simulink model "TVModel_2022"  (R2022a)
settings: Solver=FixedStepDiscrete  StartTime=0.0  StopTime=10.0  FixedStep=0.01  MaxStep=0.01  RelTol=1e-3  EnableMultiTasking=on
undefined symbols (not defined in the file or in its folder): TV
libraries: simulink x5, simulink_extras x4, dspstat3 x2, sharedTrackingLibrary x1, slpidlib x1, eeGeneralControl x1
(part 1 of 4)
settings Model: Creator=giuse  LastModifiedBy=Daniele
settings SolverCC: AutoInsertRateTranBlk=on
settings OptimizationCC: DefaultParameterBehavior=Inlined  UseDivisionForNetSlopeComputation=on  GainParamInheritBuiltInType=on  UseFloatMulNetSlope=on  InlineInvariantSignals=on  PassReuseOutputArgsAs=Individual arguments  ZeroExternalMemoryAtStartup=off  ZeroInternalMemoryAtStartup=off  NoFixptDivByZeroProtection=on  EfficientFloat2IntCast=on  LifeSpan=1  OptimizeBlockOrder=speed  DifferentSizesBufferReuse=on  EfficientTunableParamExpr=on
settings DebuggingCC: ParameterTunabilityLossMsg=error  UnconnectedInputMsg=warning  UnconnectedOutputMsg=warning  UnconnectedLineMsg=warning
settings HardwareCC: ProdBitPerPointer=32  ProdBitPerSizeT=32  ProdBitPerPtrDiffT=32  ProdLargestAtomicInteger=Long  ProdLargestAtomicFloat=Double  ProdWordSize=32  ProdLongLongMode=on  ProdHWDeviceType=ARM Compatible->ARM Cortex-M
settings SFSimCC: SimCustomHeaderCode="#include \"ITB_Nucleo_configuration\\Inc\\acados_wrapper.h\""  SimUserSources=ITB_Nucleo_configuration\Src\acados_wrapper.c  MATLABDynamicMemAlloc=off  CustomCodeUndefinedFunction=DoNotDetect
settings RTWCC: SystemTargetFile=ert.tlc  GenCodeOnly=on  TemplateMakefile=ert_default_tmf  RTWUseSimCustomCode=on  CustomHeaderCode="#include \"ITB_Nucleo_configuration\\Inc\\acados_wrapper.h\""  CustomSource=ITB_Nucleo_configuration\Src\acados_wrapper.c  DLArmComputeVersion=19.05
settings CodeAppCC: ForceParamTrailComments=on  IgnoreCustomStorageClasses=off  OperatorAnnotations=on  SimulinkDataObjDesc=on  SFDataObjDesc=on  CustomSymbolStrGlobalVar=rt$N$M  CustomSymbolStrType=$N$M  CustomSymbolStrFcn=$N$M$F  CustomSymbolStrMacro=$N$M  InsertBlockDesc=on
settings ERTTargetCC: TargetLangStandard=C99 (ISO)  GenerateSampleERTMain=on  IncludeMdlTerminateFcn=off  CombineSignalStateStructs=on  SuppressErrorStatus=on  SupportAbsoluteTime=off  SupportComplex=off  InlinedParameterPlacement=NonHierarchical  ERTCustomFileTemplate=example_file_process.tlc  ERTFilePackagingFormat=CompactWithDataFile

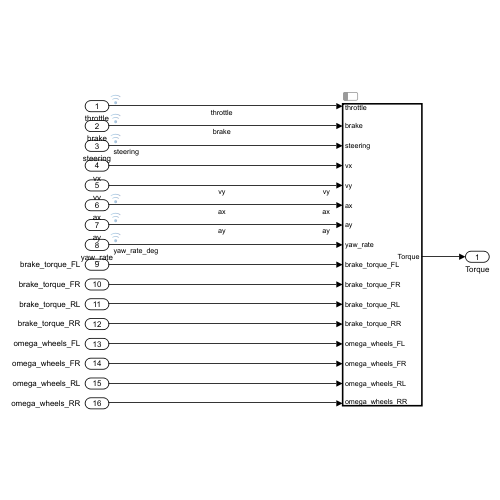
[thumbnail: Simulink's stored preview of the top-level diagram]
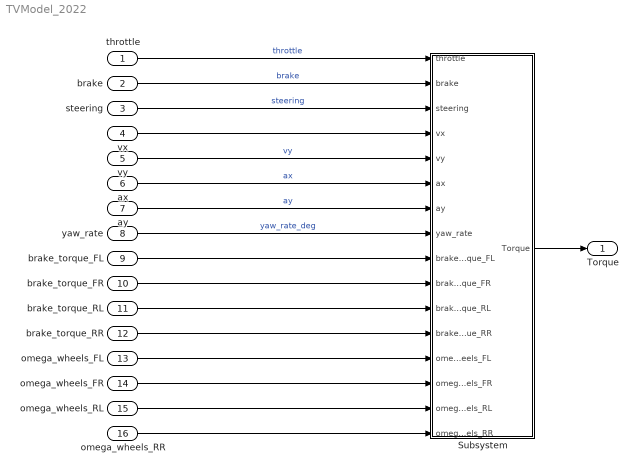
== system TVModel_2022 ==
  throttle : Inport  PortDimensions=1
  brake : Inport  Port=2  PortDimensions=1
  steering : Inport  Port=3  PortDimensions=1
  vx : Inport  Port=4  PortDimensions=1
  vy : Inport  Port=5  PortDimensions=1
  ax : Inport  Port=6  PortDimensions=1
  ay : Inport  Port=7  PortDimensions=1
  yaw_rate : Inport  Port=8  PortDimensions=1
  brake_torque_FL : Inport  Port=9  PortDimensions=1
  brake_torque_FR : Inport  Port=10  PortDimensions=1
  brake_torque_RL : Inport  Port=11  PortDimensions=1
  brake_torque_RR : Inport  Port=12  PortDimensions=1
  omega_wheels_FL : Inport  Port=13  PortDimensions=1
  omega_wheels_FR : Inport  Port=14  PortDimensions=1
  omega_wheels_RL : Inport  Port=15  PortDimensions=1
  omega_wheels_RR : Inport  Port=16  PortDimensions=1
  Subsystem : Subsystem  TreatAsAtomicUnit=on  ScheduleAs=Periodic partition  PartitionName=Subsystem  SystemSampleTime=0.02
  Torque : Outport
  wires:
  vy/1 -> Subsystem/5(vy)  "vy"
  ax/1 -> Subsystem/6(ax)  "ax"
  brake/1 -> Subsystem/2(brake)  "brake"
  ay/1 -> Subsystem/7(ay)  "ay"
  brake_torque_RL/1 -> Subsystem/11(brake_torque_RL)
  brake_torque_RR/1 -> Subsystem/12(brake_torque_RR)
  omega_wheels_RR/1 -> Subsystem/16(omega_wheels_RR)
  omega_wheels_FL/1 -> Subsystem/13(omega_wheels_FL)
  brake_torque_FR/1 -> Subsystem/10(brake_torque_FR)
  yaw_rate/1 -> Subsystem/8(yaw_rate)  "yaw_rate_deg"
  omega_wheels_FR/1 -> Subsystem/14(omega_wheels_FR)
  omega_wheels_RL/1 -> Subsystem/15(omega_wheels_RL)
  steering/1 -> Subsystem/3(steering)  "steering"
  brake_torque_FL/1 -> Subsystem/9(brake_torque_FL)
  vx/1 -> Subsystem/4(vx)
  throttle/1 -> Subsystem/1(throttle)  "throttle"
  Subsystem/1(Torque) -> Torque/1

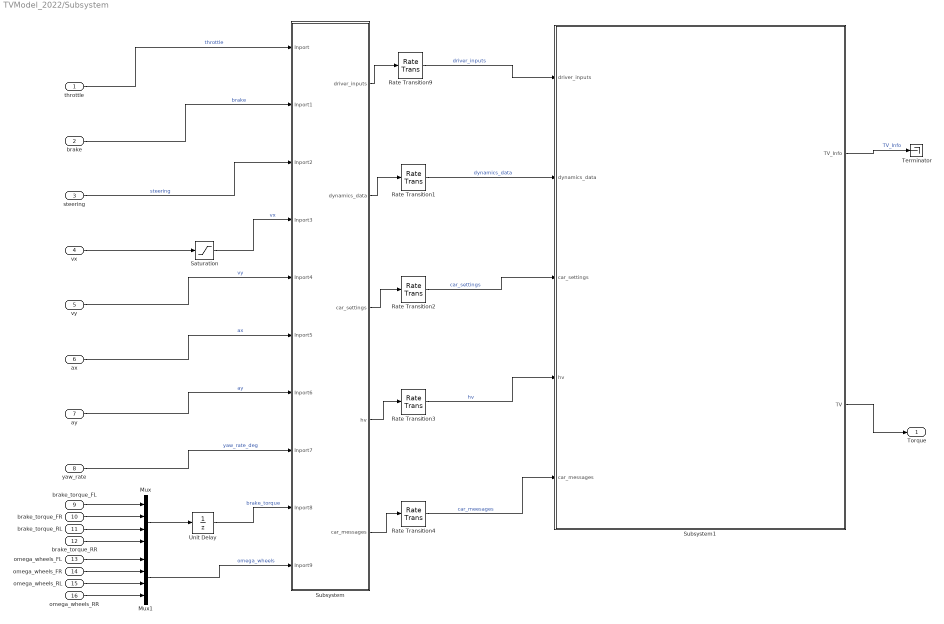
== system TVModel_2022/Subsystem ==
  throttle : Inport
  brake : Inport  Port=2
  steering : Inport  Port=3
  vx : Inport  Port=4
  vy : Inport  Port=5
  ax : Inport  Port=6
  ay : Inport  Port=7
  yaw_rate : Inport  Port=8
  brake_torque_FL : Inport  Port=9
  brake_torque_FR : Inport  Port=10
  brake_torque_RL : Inport  Port=11
  brake_torque_RR : Inport  Port=12
  omega_wheels_FL : Inport  Port=13
  omega_wheels_FR : Inport  Port=14
  omega_wheels_RL : Inport  Port=15
  omega_wheels_RR : Inport  Port=16
  Mux : Mux
  Mux1 : Mux
  Rate Transition{1..4,9} (5 alike) : RateTransition  OutPortSampleTime=TV.MPC.T/TV.MPC.N
  Saturation : Saturate  UpperLimit=inf  LowerLimit=0
  Subsystem : Subsystem
  Subsystem1 : Subsystem
  Terminator : Terminator
  Unit Delay : UnitDelay  SampleTime=-1  HasFrameUpgradeWarning=on
  Torque : Outport
  wires:
  omega_wheels_FL/1 -> Mux1/1
  ax/1 -> Subsystem/6(Inport5)  "ax"
  Unit Delay/1 -> Subsystem/9(Inport8)  "brake_torque"
  vy/1 -> Subsystem/5(Inport4)  "vy"
  ay/1 -> Subsystem/7(Inport6)  "ay"
  Mux1/1 -> Subsystem/10(Inport9)  "omega_wheels"
  Saturation/1 -> Subsystem/4(Inport3)  "vx"
  brake/1 -> Subsystem/2(Inport1)  "brake"
  yaw_rate/1 -> Subsystem/8(Inport7)  "yaw_rate_deg"
  throttle/1 -> Subsystem/1(Inport)  "throttle"
  brake_torque_RL/1 -> Mux/3
  vx/1 -> Saturation/1
  brake_torque_FL/1 -> Mux/1
  omega_wheels_RR/1 -> Mux1/4
  brake_torque_RR/1 -> Mux/4
  steering/1 -> Subsystem/3(Inport2)  "steering"
  omega_wheels_FR/1 -> Mux1/2
  Mux/1 -> Unit Delay/1
  omega_wheels_RL/1 -> Mux1/3
  brake_torque_FR/1 -> Mux/2
  Subsystem1/2(TV) -> Torque/1
  Subsystem/1(driver_inputs) -> Rate Transition9/1
  Rate Transition2/1 -> Subsystem1/3(car_settings)  "car_settings"
  Rate Transition1/1 -> Subsystem1/2(dynamics_data)  "dynamics_data"
  Rate Transition3/1 -> Subsystem1/4(hv)  "hv"
  Subsystem/2(dynamics_data) -> Rate Transition1/1
  Subsystem/5(car_messages) -> Rate Transition4/1
  Rate Transition4/1 -> Subsystem1/5(car_messages)  "car_meesages"
  Subsystem/4(hv) -> Rate Transition3/1
  Subsystem/3(car_settings) -> Rate Transition2/1
  Rate Transition9/1 -> Subsystem1/1(driver_inputs)  "driver_inputs"
  Subsystem1/1(TV_Info) -> Terminator/1  "TV_Info"

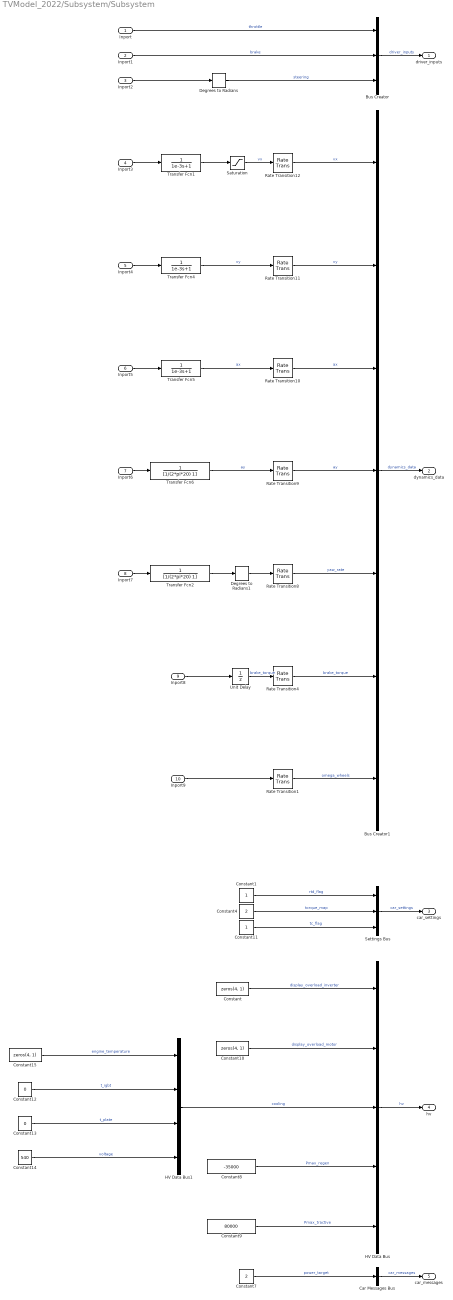
== system TVModel_2022/Subsystem/Subsystem ==
  Inport : Inport
  Inport1 : Inport  Port=2
  Inport2 : Inport  Port=3
  Inport3 : Inport  Port=4
  Inport4 : Inport  Port=5
  Inport5 : Inport  Port=6
  Inport6 : Inport  Port=7
  Inport7 : Inport  Port=8
  Inport8 : Inport  Port=9
  Inport9 : Inport  Port=10
  Bus Creator : BusCreator  Inputs=3
  Bus Creator1 : BusCreator  Inputs=7
  Car Messages Bus : BusCreator  Inputs=1
  Constant : Constant  Value=zeros(4, 1)
  Constant1 : Constant  OutDataTypeStr=uint8
  Constant10 : Constant  Value=zeros(4, 1)
  Constant11 : Constant  OutDataTypeStr=uint8
  Constant12 : Constant  Value=0
  Constant13 : Constant  Value=0
  Constant14 : Constant  Value=540
  Constant15 : Constant  Value=zeros(4, 1)
  Constant4 : Constant  Value=2  OutDataTypeStr=uint8
  Constant7 : Constant  Value=2
  Constant8 : Constant  Value=-35000
  Constant9 : Constant  Value=80000
  Degrees to Radians : simulink_extras/Transformations/Degrees to Radians
  Degrees to Radians1 : simulink_extras/Transformations/Degrees to Radians
  HV Data Bus : BusCreator  Inputs=5
  HV Data Bus1 : BusCreator  Inputs=4
  Rate Transition{1,4,8..12} (7 alike) : RateTransition  OutPortSampleTime=0.001
  Saturation : Saturate  UpperLimit=inf  LowerLimit=0
  Settings Bus : BusCreator  Inputs=3
  Transfer Fcn1 : TransferFcn  Denominator=[1e-3 1]
  Transfer Fcn2 : TransferFcn  Denominator=[1/(2*pi*20) 1]
  Transfer Fcn4 : TransferFcn  Denominator=[1e-3 1]
  Transfer Fcn5 : TransferFcn  Denominator=[1e-3 1]
  Transfer Fcn6 : TransferFcn  Denominator=[1/(2*pi*20) 1]
  Unit Delay : UnitDelay  SampleTime=-1  HasFrameUpgradeWarning=on
  driver_inputs : Outport
  dynamics_data : Outport  Port=2
  car_settings : Outport  Port=3
  hv : Outport  Port=4
  car_messages : Outport  Port=5
  wires:
  Constant10/1 -> HV Data Bus/2  "display_overload_motor"
  Constant4/1 -> Settings Bus/2  "torque_map"
  Rate Transition4/1 -> Bus Creator1/6  "brake_torque"
  Degrees to Radians/1 -> Bus Creator/3  "steering"
  Constant1/1 -> Settings Bus/1  "rtd_flag"
  Car Messages Bus/1 -> car_messages/1  "car_messages"
  Rate Transition1/1 -> Bus Creator1/7  "omega_wheels"
  Rate Transition9/1 -> Bus Creator1/4  "ay"
  Constant/1 -> HV Data Bus/1  "display_overload_inverter"
  Rate Transition10/1 -> Bus Creator1/3  "ax"
  Rate Transition8/1 -> Bus Creator1/5  "yaw_rate"
  Degrees to Radians1/1 -> Rate Transition8/1
  Rate Transition11/1 -> Bus Creator1/2  "vy"
  Constant7/1 -> Car Messages Bus/1  "power_target"
  Rate Transition12/1 -> Bus Creator1/1  "vx"
  Bus Creator/1 -> driver_inputs/1  "driver_inputs"
  Inport2/1 -> Degrees to Radians/1
  Transfer Fcn2/1 -> Degrees to Radians1/1
  HV Data Bus/1 -> hv/1  "hv"
  Settings Bus/1 -> car_settings/1  "car_settings"
  Bus Creator1/1 -> dynamics_data/1  "dynamics_data"
  Constant8/1 -> HV Data Bus/4  "Pmax_regen"
  Constant9/1 -> HV Data Bus/5  "Pmax_tractive"
  Constant11/1 -> Settings Bus/3  "tc_flag"
  Constant15/1 -> HV Data Bus1/1  "engine_temperature"
  Constant14/1 -> HV Data Bus1/4  "voltage"
  Constant13/1 -> HV Data Bus1/3  "t_plate"
  HV Data Bus1/1 -> HV Data Bus/3  "cooling"
  Constant12/1 -> HV Data Bus1/2  "t_igbt"
  Transfer Fcn6/1 -> Rate Transition9/1  "ay"
  Transfer Fcn5/1 -> Rate Transition10/1  "ax"
  Transfer Fcn4/1 -> Rate Transition11/1  "vy"
  Inport7/1 -> Transfer Fcn2/1
  Inport/1 -> Bus Creator/1  "throttle"
  Inport6/1 -> Transfer Fcn6/1
  Inport4/1 -> Transfer Fcn4/1
  Unit Delay/1 -> Rate Transition4/1  "brake_torque"
  Inport8/1 -> Unit Delay/1
  Inport1/1 -> Bus Creator/2  "brake"
  Inport3/1 -> Transfer Fcn1/1
  Saturation/1 -> Rate Transition12/1  "vx"
  Inport5/1 -> Transfer Fcn5/1
  Transfer Fcn1/1 -> Saturation/1
  Inport9/1 -> Rate Transition1/1

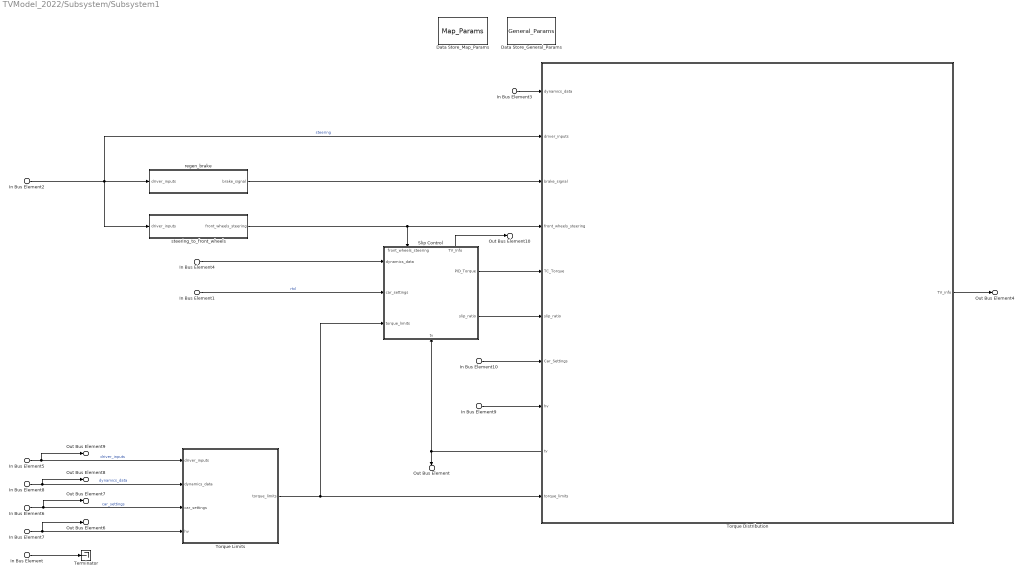
== system TVModel_2022/Subsystem/Subsystem1 ==
  In Bus Element2 : Inport  PortName=driver_inputs
  In Bus Element5 : Inport  PortName=driver_inputs
  In Bus Element3 : Inport  Port=2  PortName=dynamics_data
  In Bus Element4 : Inport  Port=2  PortName=dynamics_data
  In Bus Element8 : Inport  Port=2  PortName=dynamics_data
  In Bus Element6 : Inport  Port=3  PortName=car_settings
  In Bus Element10 : Inport  Port=3  PortName=car_settings
  In Bus Element1 : Inport  Port=3  PortName=car_settings
  In Bus Element7 : Inport  Port=4  PortName=hv
  In Bus Element9 : Inport  Port=4  PortName=hv
  In Bus Element : Inport  Port=5  PortName=car_messages
  Data Store_General_Params : DataStoreMemory  DataStoreName=General_Params  WriteAfterWriteMsg=warning  WriteAfterReadMsg=warning  InitialValue=TV.LV.GENERAL  ShowAdditionalParam=off  OutDataTypeStr=Bus: zGeneral_Params
  Data Store_Map_Params : DataStoreMemory  DataStoreName=Map_Params  WriteAfterWriteMsg=warning  WriteAfterReadMsg=warning  InitialValue=TV.LV.MAP  ShowAdditionalParam=off  OutDataTypeStr=Bus: zMap_Params
  Slip Control : Subsystem
      settings: PortSchema="{\"entries\":[{\"content\":{\"sides\":[{\"content\":{\"connectorIds\":[\"In1\",\"In2\",\"In3\"]},\"type\":\"ConnectorPlacement.EquallySpacedRectSide\",\"uuid\":\"8a9d1e07-b328-4196-9b4d-e7b80486ea0d\"},{\"content\":{\"connectorIds\":[\"Out1\",\"Out2\"],\"side\":\"RIGHT\"},\"type\":\"ConnectorPlacement.EquallySpacedRectSide\",\"uuid\":\"54b02848-08e3-4b14-88b1-ac4e3b76af35\"},{\"content\":{\"connectorIds\":[\"In4\",\"Out3\"],\"side\":\"TOP\"},\"type\":\"ConnectorPlacement.EquallySpacedRectSide\",\"uuid\":\"fa58ad84-8b37-4040-ab0d-44b4a46d9cd3\"},{\"content\":{\"connectorIds\":[\"In5\"],\"side\":\"BOTTOM\"},\"type\":\"ConnectorPlacement.EquallySpacedRectSide\",\"uuid\":\"9f701fac-df9e-44a7-8b60-14e13ec38994\"}]},\"type\":\"ConnectorPlacement.EquallySpacedConnector\",\"uuid\":\"79668f27-9637-4f32-93ba-543b2692eb5a\"}],\"packageUris\":[\"http://schema.mathworks.com/mf0/Connector/R2020b\"],\"version\":\"1.0\"}"
      mask Display: image('$imagefile'); % Use "Edit Image" on toolstrip to change.
  Terminator : Terminator
  Torque Distribution : Subsystem
      settings: PortSchema="{\"entries\":[{\"content\":{\"sides\":[{\"content\":{\"connectorIds\":[\"In1\",\"In2\",\"In3\",\"In4\",\"In5\",\"In6\",\"In7\",\"In8\",\"Out2\",\"In9\"]},\"type\":\"ConnectorPlacement.EquallySpacedRectSide\",\"uuid\":\"8028a4c9-ddd7-4405-9e82-68c07343a662\"},{\"content\":{\"connectorIds\":[\"Out1\"],\"side\":\"RIGHT\"},\"type\":\"ConnectorPlacement.EquallySpacedRectSide\",\"uuid\":\"bb85ae62-6999-48a4-8d6f-4b5feb08430d\"},{\"content\":{\"connectorIds\":[],\"side\":\"TOP\"},\"type\":\"ConnectorPlacement.EquallySpacedRectSide\",\"uuid\":\"2aeaf336-9fee-4907-aa0d-838f403ef7c5\"}]},\"type\":\"ConnectorPlacement.EquallySpacedConnector\",\"uuid\":\"30067ecc-f7ce-4215-a9f2-43b0c1069aa3\"}],\"packageUris\":[\"http://schema.mathworks.com/mf0/Connector/R2020b\"],\"version\":\"1.0\"}"
      mask Display: image('$imagefile'); % Use "Edit Image" on toolstrip to change.
  Torque Limits : Subsystem
      mask Display: image('$imagefile'); % Use "Edit Image" on toolstrip to change.
  regen_brake : Subsystem
  steering_to_front_wheels : Subsystem
  Out Bus Element4 : Outport  PortName=TV_Info  Element=Torque_Distribution
  Out Bus Element6 : Outport  PortName=TV_Info  Element=Input_Signals.hv
  Out Bus Element7 : Outport  PortName=TV_Info  Element=Input_Signals.car_settings
  Out Bus Element8 : Outport  PortName=TV_Info  Element=Input_Signals.dynamics_data
  Out Bus Element9 : Outport  PortName=TV_Info  Element=Input_Signals.driver_inputs
  Out Bus Element10 : Outport  PortName=TV_Info  Element=Slip_Control
  Out Bus Element : Outport  Port=2  PortName=TV
  wires:
  steering_to_front_wheels/1(front_wheels_steering) -> Torque Distribution/4(front_wheels_steering), Slip Control/4(front_wheels_steering)
  In Bus Element7/1 -> Out Bus Element6/1, Torque Limits/4(hv)
  Torque Distribution/1(TV_info) -> Out Bus Element4/1
  In Bus Element1/1 -> Slip Control/2(car_settings)  "rtd"
  In Bus Element8/1 -> Torque Limits/2(dynamics_data), Out Bus Element8/1  "dynamics_data"
  In Bus Element2/1 -> steering_to_front_wheels/1(driver_inputs), regen_brake/1(driver_inputs), Torque Distribution/2(driver_inputs)  "steering"
  In Bus Element9/1 -> Torque Distribution/8(hv)
  In Bus Element5/1 -> Torque Limits/1(driver_inputs), Out Bus Element9/1  "driver_inputs"
  In Bus Element6/1 -> Out Bus Element7/1, Torque Limits/3(car_settings)  "car_settings"
  Slip Control/1(PID_Torque) -> Torque Distribution/5(TC_Torque)
  Torque Limits/1(torque_limits) -> Slip Control/3(torque_limits), Torque Distribution/9(torque_limits)
  In Bus Element10/1 -> Torque Distribution/7(Car_Settings)
  Slip Control/3(TV_Info) -> Out Bus Element10/1
  In Bus Element/1 -> Terminator/1
  regen_brake/1(brake_signal) -> Torque Distribution/3(brake_signal)
  Slip Control/2(slip_ratio) -> Torque Distribution/6(slip_ratio)
  Torque Distribution/2(tv) -> Out Bus Element/1, Slip Control/5(tv)
  In Bus Element4/1 -> Slip Control/1(dynamics_data)
  In Bus Element3/1 -> Torque Distribution/1(dynamics_data)

== system TVModel_2022/Subsystem/Subsystem1/Slip Control ==
  In Bus Element1 : Inport  PortName=dynamics_data
  In Bus Element2 : Inport  Port=2  PortName=car_settings
  In Bus Element : Inport  Port=3  PortName=torque_limits
  In Bus Element6 : Inport  Port=4  PortName=front_wheels_steering
  In Bus Element7 : Inport  Port=5  PortName=tv
  Slip Ratios : Subsystem
  Traction_PID : Subsystem  Commented=on
  Out Bus Element1 : Outport  PortName=PID_Torque
  Out Bus Element : Outport  Port=2  PortName=slip_ratio
  Out Bus Element7 : Outport  Port=3  PortName=TV_Info  Element=Slip_Ratios
  wires:
  Slip Ratios/1(slip_ratio) -> Traction_PID/4(slip_ratio), Out Bus Element/1  "slip_ratio"
  In Bus Element1/1 -> Slip Ratios/1(dynamics_data)  "dynamics_data"
  In Bus Element6/1 -> Slip Ratios/2(front_wheels_steering)
  Slip Ratios/2(TV_Info) -> Out Bus Element7/1
  Traction_PID/1(PID_Torque) -> Out Bus Element1/1
  In Bus Element2/1 -> Traction_PID/2(car_settings)  "rtd"
  In Bus Element/1 -> Traction_PID/3(torque_limits)  "t_limit_positive"
  In Bus Element7/1 -> Traction_PID/1(tv)

== system TVModel_2022/Subsystem/Subsystem1/Torque Distribution ==
  In Bus Element : Inport  PortName=dynamics_data
  In Bus Element1 : Inport  Port=2  PortName=driver_inputs
  In Bus Element3 : Inport  Port=3  PortName=brake_signal
  In Bus Element2 : Inport  Port=4  PortName=front_wheels_steering
  In Bus Element6 : Inport  Port=4  PortName=front_wheels_steering
  In Bus Element7 : Inport  Port=5  PortName=TC_Torque
  In Bus Element5 : Inport  Port=6  PortName=slip_ratio
  In Bus torque_map : Inport  Port=7  PortName=Car_Settings
  In Bus Element8 : Inport  Port=8  PortName=hv
  In Bus Element4 : Inport  Port=9  PortName=torque_limits
  MPC : Subsystem
      mask Display: image('$imagefile'); % Use "Edit Image" on toolstrip to change.
  Reference Tracking : Subsystem
      mask Display: image('$imagefile'); % Use "Edit Image" on toolstrip to change.
  Out Bus Element1 : Outport  PortName=TV_info  Element=MPC
  Out Bus Element : Outport  PortName=TV_info  Element=Reference
  Out Bus Element18 : Outport  Port=2  PortName=tv
  wires:
  In Bus torque_map/1 -> MPC/9(Car_Setting)
  In Bus Element5/1 -> MPC/4(slip_ratio)
  In Bus Element4/1 -> MPC/1(mpc_torque_limit)  "torque_limits_signals"
  In Bus Element3/1 -> MPC/7(brake_signal)  "regen"
  In Bus Element2/1 -> MPC/6(front_wheel_angles)  "front_wheels_steering_signals"
  Reference Tracking/2(yaw_rate_desired) -> MPC/3(yaw_rate_desired)  "yaw_rate_desired"
  In Bus Element/1 -> MPC/2(dynamics_data), Reference Tracking/1(dynamics_data)
  In Bus Element1/1 -> MPC/5(driver_inputs)  "driver_inputs_signals"
  In Bus Element6/1 -> Reference Tracking/2(front_wheels_steering)
  Reference Tracking/1(TV_Info) -> Out Bus Element/1
  MPC/1(TV_Info) -> Out Bus Element1/1
  In Bus Element7/1 -> MPC/8(TC_Torque)
  In Bus Element8/1 -> MPC/10(hv)  "hv"
  MPC/2(TV) -> Out Bus Element18/1

== system TVModel_2022/Subsystem/Subsystem1/Torque Limits ==
  In Bus throttle : Inport  PortName=driver_inputs
  In Bus Element6 : Inport  Port=2  PortName=dynamics_data
  In Bus Element3 : Inport  Port=2  PortName=dynamics_data
  In Bus torque_map1 : Inport  Port=3  PortName=car_settings
  In Bus torque_map3 : Inport  Port=3  PortName=car_settings
  In Bus torque_map2 : Inport  Port=3  PortName=car_settings
  In Bus Element2 : Inport  Port=4  PortName=hv
  In Bus Element1 : Inport  Port=4  PortName=hv
  Torque Limits Positive : Subsystem
      mask Display: image('$imagefile'); % Use "Edit Image" on toolstrip to change.
  Torque Limits Regen : Subsystem
      mask Display: image('$imagefile'); % Use "Edit Image" on toolstrip to change.
  Torque Request : Subsystem
      mask Display: image('$imagefile'); % Use "Edit Image" on toolstrip to change.
  Out Bus Element : Outport  PortName=torque_limits  Element=t_req
  Out Bus Element2 : Outport  PortName=torque_limits  Element=t_limit_positive
  Out Bus Element4 : Outport  PortName=torque_limits  Element=t_limit_negative
  wires:
  Torque Limits Regen/1(t_limit_regen) -> Out Bus Element4/1  "t_limit_negative"
  Torque Limits Positive/1(t_limit_positive) -> Out Bus Element2/1
  Torque Request/1(t_req) -> Out Bus Element/1
  In Bus throttle/1 -> Torque Request/1(driver_inputs)  "throttle"
  In Bus torque_map3/1 -> Torque Request/2(Car_Settings)  "torque_map"
  In Bus Element2/1 -> Torque Limits Positive/2(hv)  "hv"
  In Bus Element6/1 -> Torque Limits Positive/3(dynamics_data)  "omega_wheels"
  In Bus torque_map1/1 -> Torque Limits Positive/1(car_settings)  "torque_map"
  In Bus torque_map2/1 -> Torque Limits Regen/1(car_settings)  "torque_map"
  In Bus Element1/1 -> Torque Limits Regen/2(hv)  "hv"
  In Bus Element3/1 -> Torque Limits Regen/3(dynamics_data)  "omega_wheels"

== system TVModel_2022/Subsystem/Subsystem1/regen_brake ==
  In Bus Element : Inport  PortName=driver_inputs  Element=brake
  Gain : Gain  Gain=1/0.28
  Saturation : Saturate  UpperLimit=1  LowerLimit=0
  Out Bus Element : Outport  PortName=brake_signal  Element=regen
  wires:
  Gain/1 -> Saturation/1
  In Bus Element/1 -> Gain/1
  Saturation/1 -> Out Bus Element/1

== system TVModel_2022/Subsystem/Subsystem1/steering_to_front_wheels ==
  In Bus Element : Inport  PortName=driver_inputs  Element=steering
  In Bus Element1 : Inport  PortName=driver_inputs  Element=steering
  Abs : Abs  SaturateOnIntegerOverflow=off
  Divide1 : Product  Inputs=**
  Mux : Mux  Inputs=2
  Sign : Signum
  Unary Minus : UnaryMinus
  steering_to_wheel_angle_single_axis_LUT : Lookup_n-D  NumberOfTableDimensions=1  BreakpointsForDimension1=TV.LUT.Car_LUT.steer_at_ground_single_axis_LUT.Steering  Table=TV.LUT.Car_LUT.steer_at_ground_single_axis_LUT.SteerAngle_SingleAxis  InternalRulePriority=Speed  RndMeth=Simplest
  steering_to_wheel_angles_LUT : Lookup_n-D  NumberOfTableDimensions=1  BreakpointsForDimension1=TV.LUT.Car_LUT.steer_at_ground_LUT.Steering  Table=TV.LUT.Car_LUT.steer_at_ground_LUT.SteerAngle_FL  InternalRulePriority=Speed  RndMeth=Simplest
  Out Bus Element : Outport  PortName=front_wheels_steering  Element=single_axis
  Out Bus Element1 : Outport  PortName=front_wheels_steering  Element=different_axis
  wires:
  Divide1/1 -> Out Bus Element1/1  "front_wheel_angle_single_axis_different_axis"
  steering_to_wheel_angle_single_axis_LUT/1 -> Out Bus Element/1  "front_wheel_angle_single_axis"
  Sign/1 -> Divide1/2
  Unary Minus/1 -> Mux/2
  In Bus Element/1 -> steering_to_wheel_angle_single_axis_LUT/1
  steering_to_wheel_angles_LUT/1 -> Abs/1  "front_wheel_angles"
  Mux/1 -> steering_to_wheel_angles_LUT/1
  Abs/1 -> Divide1/1
  In Bus Element1/1 -> Sign/1, Mux/1, Unary Minus/1

== system TVModel_2022/Subsystem/Subsystem1/Slip Control/Slip Ratios ==
  In Bus Element{,2,4..5} (4 alike) : Inport  PortName=dynamics_data
  In Bus Element6 : Inport  Port=2  PortName=front_wheels_steering
  In Bus Element1 : Inport  Port=2  PortName=front_wheels_steering
  FL SR : Subsystem
  FR SR : Subsystem
  "RL RR " : Subsystem
  RL SR : Subsystem
  Out Bus Element : Outport  PortName=slip_ratio  Element=fl
  Out Bus Element1 : Outport  PortName=slip_ratio  Element=fr
  Out Bus Element2 : Outport  PortName=slip_ratio  Element=rl
  Out Bus Element3 : Outport  PortName=slip_ratio  Element=rr
  Out Bus Element4 : Outport  Port=2  PortName=TV_Info  Element=slip_ratio_fl
  Out Bus Element5 : Outport  Port=2  PortName=TV_Info  Element=slip_ratio_fr
  Out Bus Element6 : Outport  Port=2  PortName=TV_Info  Element=slip_ratio_rl
  Out Bus Element7 : Outport  Port=2  PortName=TV_Info  Element=slip_ratio_rr
  wires:
  In Bus Element5/1 -> "RL RR "/1(dynamics_data)
  In Bus Element4/1 -> RL SR/1(dynamics_data)
  In Bus Element2/1 -> FR SR/1(dynamics_data)
  In Bus Element1/1 -> FR SR/2(front_wheels_steering)
  In Bus Element6/1 -> FL SR/2(front_wheels_steering)
  In Bus Element/1 -> FL SR/1(dynamics_data)
  "RL RR "/1(RR) -> Out Bus Element7/1, Out Bus Element3/1  "kappa_RR"
  FR SR/1(FR) -> Out Bus Element5/1, Out Bus Element1/1  "kappa_FR"
  FL SR/1(FL) -> Out Bus Element4/1, Out Bus Element/1  "kappa_FL"
  RL SR/1(RL) -> Out Bus Element6/1, Out Bus Element2/1  "kappa_RL"

== system TVModel_2022/Subsystem/Subsystem1/Slip Control/Traction_PID ==
  In Bus Element7 : Inport  PortName=tv
  In Bus Element6 : Inport  Port=2  PortName=car_settings  Element=rtd_flag
  In Bus Element5 : Inport  Port=2  PortName=car_settings  Element=tc_flag
  In Bus Element : Inport  Port=3  PortName=torque_limits  Element=t_limit_positive
  Bus Element In5 : Inport  Port=4  PortName=slip_ratio
  Bus Element In6 : Inport  Port=4  PortName=slip_ratio
  Constant17 : Constant  Value=0.1
  Constant18 : Constant  Value=10e-3
  Constant19 : Constant  Value=0.001
  Constant20 : Constant
  Constant21 : Constant  Value=0.2
  Saturation : Saturate  UpperLimit=22  LowerLimit=0
  TC : MATLAB Function  TreatAsAtomicUnit=on
  TC_Activation_Logic : Stateflow chart  TreatAsAtomicUnit=on
  Unit Delay : UnitDelay  SampleTime=-1  HasFrameUpgradeWarning=on
  Out Bus Element1 : Outport  PortName=PID_Torque
  wires:
  In Bus Element/1 -> TC_Activation_Logic/5(t_limit_positive)  "t_limit_positive"
  TC_Activation_Logic/1(t_max_pid) -> Saturation/1
  In Bus Element5/1 -> TC_Activation_Logic/4(tc_flag)  "tc_flag"
  In Bus Element6/1 -> TC_Activation_Logic/3(rtd_flag)  "rtd_flag"
  In Bus Element7/1 -> Unit Delay/1
  Bus Element In5/1 -> TC_Activation_Logic/6(slip_ratio)  "slip_ratios"
  Constant17/1 -> TC_Activation_Logic/7(slip_ratio_target)
  TC/1(t_pid) -> TC_Activation_Logic/1(t_pid)
  Constant18/1 -> TC/5(time_step)
  Constant19/1 -> TC/3(kp)
  Constant20/1 -> TC/4(ki)
  Bus Element In6/1 -> TC/2(slip_ratio)  "slip_ratios"
  Constant21/1 -> TC/1(slip_ratio_target)
  Unit Delay/1 -> TC_Activation_Logic/2(t_actual)
  Saturation/1 -> Out Bus Element1/1  "t_max_pid"

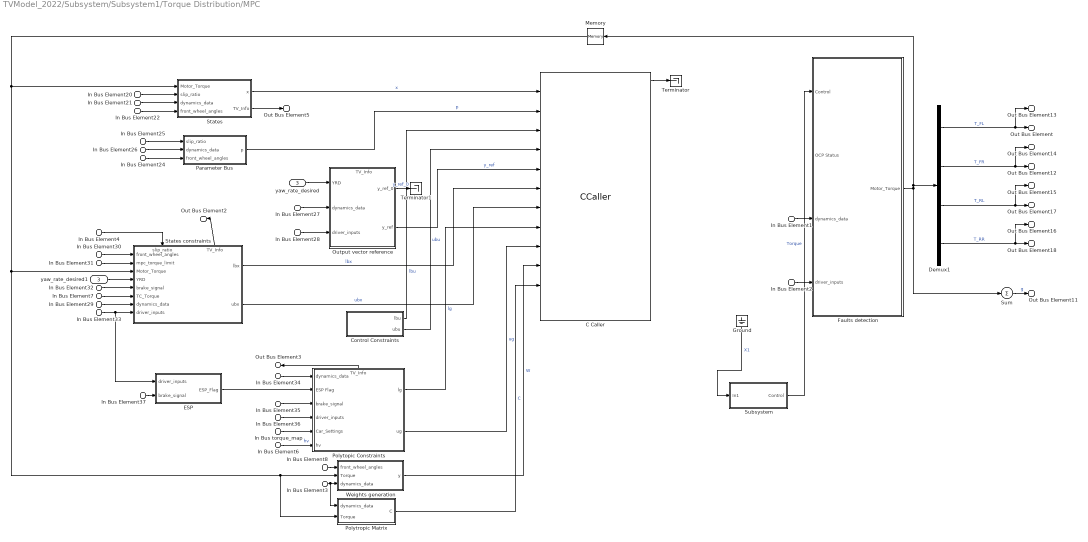
== system TVModel_2022/Subsystem/Subsystem1/Torque Distribution/MPC ==
  In Bus Element31 : Inport  PortName=mpc_torque_limit
  In Bus Element{1,3,21,26..27,29,34} (7 alike) : Inport  Port=2  PortName=dynamics_data
  yaw_rate_desired : Inport  Port=3
  In Bus Element20 : Inport  Port=4  PortName=slip_ratio
  In Bus Element25 : Inport  Port=4  PortName=slip_ratio
  In Bus Element4 : Inport  Port=4  PortName=slip_ratio
  In Bus Element{2,28,33,36} (4 alike) : Inport  Port=5  PortName=driver_inputs
  In Bus Element{8,22,24,30} (4 alike) : Inport  Port=6  PortName=front_wheel_angles
  In Bus Element32 : Inport  Port=7  PortName=brake_signal
  In Bus Element35 : Inport  Port=7  PortName=brake_signal
  In Bus Element37 : Inport  Port=7  PortName=brake_signal
  In Bus Element7 : Inport  Port=8  PortName=TC_Torque
  In Bus torque_map : Inport  Port=9  PortName=Car_Setting
  In Bus Element6 : Inport  Port=10  PortName=hv
  "     Output vector reference" : Subsystem
      settings: PortSchema="{\"entries\":[{\"content\":{\"sides\":[{\"content\":{\"connectorIds\":[\"In1\",\"In2\",\"In3\"]},\"type\":\"ConnectorPlacement.EquallySpacedRectSide\",\"uuid\":\"818c90b4-a927-40a5-b4e4-e64469099490\"},{\"content\":{\"connectorIds\":[\"Out1\",\"Out2\"],\"side\":\"RIGHT\"},\"type\":\"ConnectorPlacement.EquallySpacedRectSide\",\"uuid\":\"17c30fe6-e2a1-4832-99f1-cdba49b58b0d\"},{\"content\":{\"connectorIds\":[\"Out3\"],\"side\":\"TOP\"},\"type\":\"ConnectorPlacement.EquallySpacedRectSide\",\"uuid\":\"f76fc466-dc2c-4206-97e0-e4a76ee0f969\"}]},\"type\":\"ConnectorPlacement.EquallySpacedConnector\",\"uuid\":\"2ab2c2e2-079f-4a85-9b38-3e9c1f136cc0\"}],\"packageUris\":[\"http://schema.mathworks.com/mf0/Connector/R2020b\"],\"version\":\"1.0\"}"
  " Parameter Bus " : Subsystem
  " States" : Subsystem
  C Caller : CCaller  FunctionName=Acados_Caller_wrapper  PortSpecificationStruct="%)30     .    R!8   8    (     @         %    \"     T    !     0         %  0 \"0    $    _    07)G3F%M90  4&]R=$YA;64 4V-O<&4     26YD97@     5'EP90      4VEZ90      27-';&]B86P   X    P    !@    @    $          4    (     0    ,    !         !   P!O=70 #@   #     &    \"     0         !0    @    !     P    $         $  # &]U=  .    .     8    (    !          %    \"     $    &     0         0   ...(+7495 chars)"
  Control Constraints : Subsystem
  Demux1 : Demux
  ESP : Subsystem
  Faults detection : Subsystem
  Ground : Ground
  Memory : Memory  InheritSampleTime=on
  Polytopic Constraints : Subsystem
      settings: PortSchema="{\"entries\":[{\"content\":{\"sides\":[{\"content\":{\"connectorIds\":[\"In1\",\"In2\",\"In3\",\"In4\",\"In5\",\"In6\"]},\"type\":\"ConnectorPlacement.EquallySpacedRectSide\",\"uuid\":\"22d0c767-8026-4e61-917e-ed6448896f86\"},{\"content\":{\"connectorIds\":[\"Out1\",\"Out2\"],\"side\":\"RIGHT\"},\"type\":\"ConnectorPlacement.EquallySpacedRectSide\",\"uuid\":\"f964ddd6-6be1-423f-8a9f-d3a95ecfc059\"},{\"content\":{\"connectorIds\":[\"Out3\"],\"side\":\"TOP\"},\"type\":\"ConnectorPlacement.EquallySpacedRectSide\",\"uuid\":\"217bcf57-a9cf-49fd-8101-a16fa3add937\"}]},\"type\":\"ConnectorPlacement.EquallySpacedConnector\",\"uuid\":\"fb1e75ca-354b-4201-ad5d-403c665d994f\"}],\"packageUris\":[\"http://schema.mathworks.com/mf0/Connector/R2020b\"],\"version\":\"1.0\"}"
  Polytropic Matrix : Subsystem
  States constraints : Subsystem
      settings: PortSchema="{\"entries\":[{\"content\":{\"sides\":[{\"content\":{\"connectorIds\":[\"In1\",\"In2\",\"In3\",\"In4\",\"In5\",\"In6\",\"In7\",\"In8\"]},\"type\":\"ConnectorPlacement.EquallySpacedRectSide\",\"uuid\":\"8593e4db-af87-4ecb-ab59-e8c996123787\"},{\"content\":{\"connectorIds\":[\"Out1\",\"Out2\"],\"side\":\"RIGHT\"},\"type\":\"ConnectorPlacement.EquallySpacedRectSide\",\"uuid\":\"23cd0be0-bb8d-413f-9d07-6b27363d3732\"},{\"content\":{\"connectorIds\":[\"In9\",\"Out3\"],\"side\":\"TOP\"},\"type\":\"ConnectorPlacement.EquallySpacedRectSide\",\"uuid\":\"52595343-7562-4670-a073-f9fdd714737e\"}]},\"type\":\"ConnectorPlacement.EquallySpacedConnector\",\"uuid\":\"1e427445-f5ae-42d5-a573-15ed0b9c55e5\"}],\"packageUris\":[\"http://schema.mathworks.com/mf0/Connector/R2020b\"],\"version\":\"1.0\"}"
  Subsystem : Subsystem
  Sum : Sum  Inputs=+
  Terminator : Terminator
  Terminator1 : Terminator
  Weights generation : Subsystem
  yaw_rate_desired1 : InportShadow  Port=3
  Out Bus Element5 : Outport  PortName=TV_Info  Element=States
  Out Bus Element2 : Outport  PortName=TV_Info  Element=Control_Constraints
  Out Bus Element3 : Outport  PortName=TV_Info  Element=Polytropic Constraints
  Out Bus Element16 : Outport  PortName=TV_Info  Element=Torque.t_rr
  Out Bus Element15 : Outport  PortName=TV_Info  Element=Torque.t_rl
  Out Bus Element14 : Outport  PortName=TV_Info  Element=Torque.t_fr
  Out Bus Element13 : Outport  PortName=TV_Info  Element=Torque.t_fl
  Out Bus Element11 : Outport  PortName=TV_Info  Element=Faults.g
  Out Bus Element : Outport  Port=2  PortName=TV  Element=FL
  Out Bus Element12 : Outport  Port=2  PortName=TV  Element=FR
  Out Bus Element17 : Outport  Port=2  PortName=TV  Element=RL
  Out Bus Element18 : Outport  Port=2  PortName=TV  Element=RR
  wires:
  Subsystem/1(Control) -> Faults detection/1(Control)  "Torque"
  In Bus torque_map/1 -> Polytopic Constraints/5(Car_Settings)
  In Bus Element2/1 -> Faults detection/4(driver_inputs)
  In Bus Element1/1 -> Faults detection/3(dynamics_data)
  In Bus Element37/1 -> ESP/2(brake_signal)
  In Bus Element36/1 -> Polytopic Constraints/4(driver_inputs)
  In Bus Element35/1 -> Polytopic Constraints/3(brake_signal)
  In Bus Element34/1 -> Polytopic Constraints/1(dynamics_data)
  In Bus Element33/1 -> ESP/1(driver_inputs), States constraints/8(driver_inputs)
  In Bus Element32/1 -> States constraints/5(brake_signal)
  yaw_rate_desired1/1 -> States constraints/4(YRD)
  In Bus Element31/1 -> States constraints/2(mpc_torque_limit)
  In Bus Element30/1 -> States constraints/1(front_wheel_angles)
  In Bus Element29/1 -> States constraints/7(dynamics_data)
  In Bus Element28/1 -> "     Output vector reference"/3(driver_inputs)
  In Bus Element27/1 -> "     Output vector reference"/2(dynamics_data)
  In Bus Element24/1 -> " Parameter Bus "/3(front_wheel_angles)
  In Bus Element22/1 -> " States"/4(front_wheel_angles)
  In Bus Element26/1 -> " Parameter Bus "/2(dynamics_data)
  In Bus Element25/1 -> " Parameter Bus "/1(slip_ratio)
  In Bus Element20/1 -> " States"/2(slip_ratio)
  In Bus Element21/1 -> " States"/3(dynamics_data)
  yaw_rate_desired/1 -> "     Output vector reference"/1(YRD)
  " States"/1(x) -> C Caller/1  "x"
  ESP/1(ESP_Flag) -> Polytopic Constraints/2(ESP Flag)
  Ground/1 -> Subsystem/1(In1)  "X1"
  " Parameter Bus "/1(p) -> C Caller/2  "p"
  Sum/1 -> Out Bus Element11/1  "g"
  " States"/2(TV_Info) -> Out Bus Element5/1
  States constraints/3(TV_Info) -> Out Bus Element2/1
  Polytopic Constraints/3(TV_Info) -> Out Bus Element3/1
  Demux1/1 -> Out Bus Element/1, Out Bus Element13/1  "T_FL"
  Demux1/2 -> Out Bus Element12/1, Out Bus Element14/1  "T_FR"
  Demux1/3 -> Out Bus Element17/1, Out Bus Element15/1  "T_RL"
  Demux1/4 -> Out Bus Element18/1, Out Bus Element16/1  "T_RR"
  In Bus Element7/1 -> States constraints/6(TC_Torque)
  In Bus Element4/1 -> States constraints/9(slip_ratio)
  In Bus Element6/1 -> Polytopic Constraints/6(hv)  "hv"
  In Bus Element8/1 -> Weights generation/1(front_wheel_angles)
  In Bus Element3/1 -> Polytropic Matrix/1(dynamics_data), Weights generation/3(dynamics_data)
  Faults detection/1(Motor_Torque) -> Sum/1, Memory/1, Demux1/1
  Memory/1 -> Polytropic Matrix/2(Torque), Weights generation/2(Torque), States constraints/3(Motor_Torque), " States"/1(Motor_Torque)
  C Caller/1 -> Terminator/1
  "     Output vector reference"/2(y_ref) -> C Caller/5  "y_ref"
  "     Output vector reference"/1(y_ref_0) -> Terminator1/1  "y_ref_0"
  States constraints/2(ubx) -> C Caller/7  "ubx"
  States constraints/1(lbx) -> C Caller/6  "lbx"
  Control Constraints/1(lbu) -> C Caller/3  "lbu"
  Control Constraints/2(ubu) -> C Caller/4  "ubu"
  Polytopic Constraints/1(lg) -> C Caller/8  "lg"
  Polytopic Constraints/2(ug) -> C Caller/9  "ug"
  Weights generation/1(y) -> C Caller/10  "W"
  Polytropic Matrix/1(C) -> C Caller/11  "C"

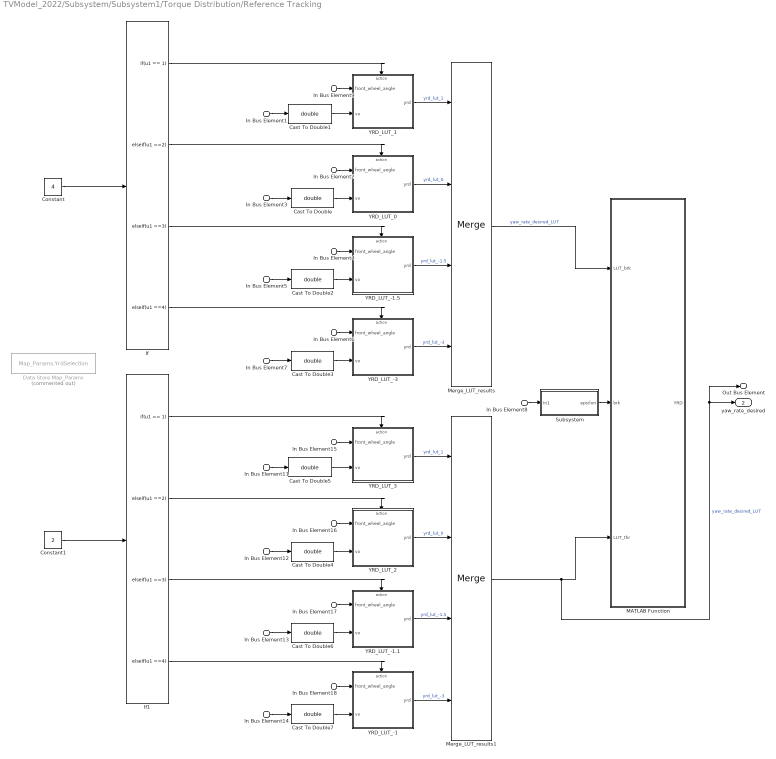
== system TVModel_2022/Subsystem/Subsystem1/Torque Distribution/Reference Tracking ==
  In Bus Element{1,3,5,7,11..14} (8 alike) : Inport  PortName=dynamics_data  Element=vx
  In Bus Element{2,4,6,8..9,15..18} (9 alike) : Inport  Port=2  PortName=front_wheels_steering  Element=single_axis
  Cast To Double{,1..7} (8 alike) : DataTypeConversion  OutDataTypeStr=double  SaturateOnIntegerOverflow=off  RndMeth=Floor
  Constant : Constant  Value=4
  Constant1 : Constant  Value=2
  Data Store Map_Params : DataStoreRead  Commented=on  DataStoreName=Map_Params  DataStoreElements=Map_Params.YrdSelection  IndexOptions=Index vector (dialog)  Indices=1  OutputSizes=1
  If : If  IfExpression=u1 == 1  ElseIfExpressions=u1 ==2,u1 ==3,u1 ==4  ShowElse=off
  If1 : If  IfExpression=u1 == 1  ElseIfExpressions=u1 ==2,u1 ==3,u1 ==4  ShowElse=off
  MATLAB Function : MATLAB Function  TreatAsAtomicUnit=on  SystemSampleTime=TV.MPC.T/TV.MPC.N
  Merge_LUT_results : Merge  Inputs=4
  Merge_LUT_results1 : Merge  Inputs=4
  Subsystem : Subsystem
  YRD_LUT_-1 : Subsystem  TreatAsAtomicUnit=on
      mask Display: image('Mask_Icon\LUT.png'); % Use "Edit Image" on toolstrip to change.
  YRD_LUT_-1.1 : Subsystem  TreatAsAtomicUnit=on
      mask Display: image('Mask_Icon\LUT.png'); % Use "Edit Image" on toolstrip to change.
  YRD_LUT_-1.5 : Subsystem  TreatAsAtomicUnit=on
      mask Display: image('Mask_Icon\LUT.png'); % Use "Edit Image" on toolstrip to change.
  YRD_LUT_-3 : Subsystem  TreatAsAtomicUnit=on
      mask Display: image('Mask_Icon\LUT.png'); % Use "Edit Image" on toolstrip to change.
  YRD_LUT_0 : Subsystem  TreatAsAtomicUnit=on
      mask Display: image('Mask_Icon\LUT.png'); % Use "Edit Image" on toolstrip to change.
  YRD_LUT_1 : Subsystem  TreatAsAtomicUnit=on
      mask Display: image('Mask_Icon\LUT.png'); % Use "Edit Image" on toolstrip to change.
  YRD_LUT_2 : Subsystem  TreatAsAtomicUnit=on
      mask Display: image('Mask_Icon\LUT.png'); % Use "Edit Image" on toolstrip to change.
  YRD_LUT_3 : Subsystem  TreatAsAtomicUnit=on
      mask Display: image('Mask_Icon\LUT.png'); % Use "Edit Image" on toolstrip to change.
  Out Bus Element : Outport  PortName=TV_Info  Element=yaw_rate_desired
  yaw_rate_desired : Outport  Port=2
  wires:
  In Bus Element9/1 -> YRD_LUT_1/1(front_wheel_angle)
  In Bus Element1/1 -> Cast To Double1/1
  In Bus Element2/1 -> YRD_LUT_0/1(front_wheel_angle)
  In Bus Element3/1 -> Cast To Double/1
  In Bus Element4/1 -> YRD_LUT_-1.5/1(front_wheel_angle)
  In Bus Element5/1 -> Cast To Double2/1
  In Bus Element6/1 -> YRD_LUT_-3/1(front_wheel_angle)
  In Bus Element7/1 -> Cast To Double3/1
  If/1 -> YRD_LUT_1/Action
  If/2 -> YRD_LUT_0/Action
  If/3 -> YRD_LUT_-1.5/Action
  If/4 -> YRD_LUT_-3/Action
  YRD_LUT_-3/1(yrd) -> Merge_LUT_results/4  "yrd_lut_-3"
  YRD_LUT_-1.5/1(yrd) -> Merge_LUT_results/3  "yrd_lut_-1.5"
  YRD_LUT_1/1(yrd) -> Merge_LUT_results/1  "yrd_lut_1"
  YRD_LUT_0/1(yrd) -> Merge_LUT_results/2  "yrd_lut_0"
  Cast To Double/1 -> YRD_LUT_0/2(vx)
  Cast To Double1/1 -> YRD_LUT_1/2(vx)
  Cast To Double2/1 -> YRD_LUT_-1.5/2(vx)
  Cast To Double3/1 -> YRD_LUT_-3/2(vx)
  Cast To Double7/1 -> YRD_LUT_-1/2(vx)
  Cast To Double6/1 -> YRD_LUT_-1.1/2(vx)
  Cast To Double5/1 -> YRD_LUT_3/2(vx)
  Cast To Double4/1 -> YRD_LUT_2/2(vx)
  YRD_LUT_2/1(yrd) -> Merge_LUT_results1/2  "yrd_lut_0"
  YRD_LUT_3/1(yrd) -> Merge_LUT_results1/1  "yrd_lut_1"
  YRD_LUT_-1.1/1(yrd) -> Merge_LUT_results1/3  "yrd_lut_-1.5"
  YRD_LUT_-1/1(yrd) -> Merge_LUT_results1/4  "yrd_lut_-3"
  If1/4 -> YRD_LUT_-1/Action
  If1/3 -> YRD_LUT_-1.1/Action
  If1/2 -> YRD_LUT_2/Action
  If1/1 -> YRD_LUT_3/Action
  In Bus Element14/1 -> Cast To Double7/1
  In Bus Element18/1 -> YRD_LUT_-1/1(front_wheel_angle)
  In Bus Element13/1 -> Cast To Double6/1
  In Bus Element17/1 -> YRD_LUT_-1.1/1(front_wheel_angle)
  In Bus Element12/1 -> Cast To Double4/1
  In Bus Element16/1 -> YRD_LUT_2/1(front_wheel_angle)
  In Bus Element11/1 -> Cast To Double5/1
  In Bus Element15/1 -> YRD_LUT_3/1(front_wheel_angle)
  Merge_LUT_results1/1 -> Out Bus Element/1, yaw_rate_desired/1, MATLAB Function/3(LUT_thr)  "yaw_rate_desired_LUT"
  Merge_LUT_results/1 -> MATLAB Function/1(LUT_brk)  "yaw_rate_desired_LUT"
  Constant/1 -> If/1
  Constant1/1 -> If1/1
  In Bus Element8/1 -> Subsystem/1(In1)
  Subsystem/1(epsilon) -> MATLAB Function/2(brk)

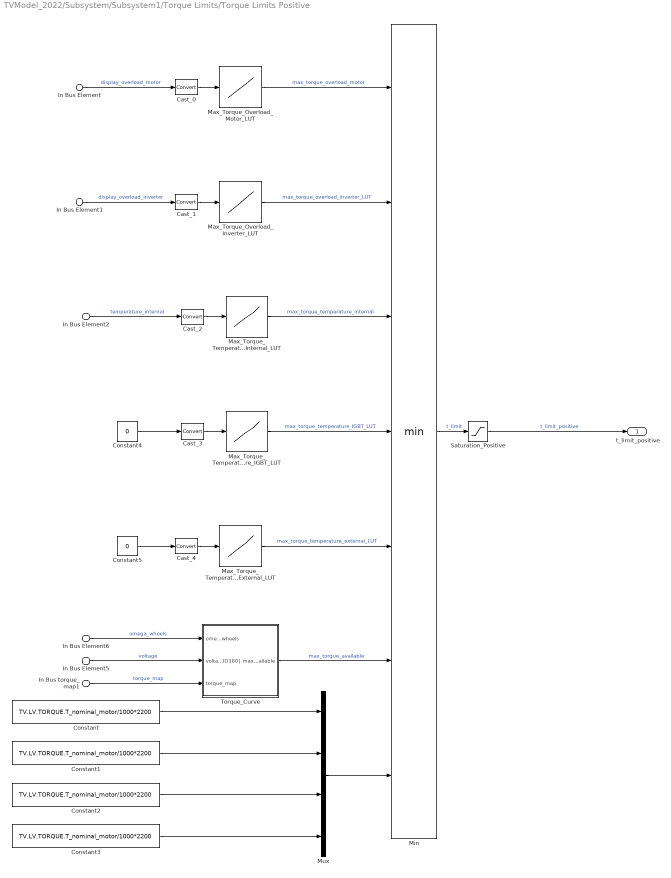
== system TVModel_2022/Subsystem/Subsystem1/Torque Limits/Torque Limits Positive ==
  In Bus torque_map1 : Inport  PortName=car_settings  Element=torque_map
  In Bus Element : Inport  Port=2  PortName=hv  Element=display_overload_motor
  In Bus Element1 : Inport  Port=2  PortName=hv  Element=display_overload_inverter
  In Bus Element2 : Inport  Port=2  PortName=hv  Element=cooling.t_plate
  In Bus Element5 : Inport  Port=2  PortName=hv  Element=cooling.voltage
  In Bus Element6 : Inport  Port=3  PortName=dynamics_data  Element=omega_wheels
  Cast_{0..4} (5 alike) : DataTypeConversion  SaturateOnIntegerOverflow=off  RndMeth=Floor
  Constant{,1..3} (4 alike) : Constant  Value=TV.LV.TORQUE.T_nominal_motor/1000*2200
  Constant4 : Constant  Value=0
  Constant5 : Constant  Value=0
  Max_Torque_Overload_Inverter_LUT : Lookup_n-D  NumberOfTableDimensions=1  BreakpointsForDimension1=[0 TV.LV.AMK.ID32999 1000]  Table=[TV.LV.AMK.ID82*TV.LV.AMK.ID32771/100 TV.LV.AMK.ID82*TV.LV.AMK.ID32771/100 0]  InternalRulePriority=Speed  RndMeth=Simplest
  Max_Torque_Overload_Motor_LUT : Lookup_n-D  NumberOfTableDimensions=1  BreakpointsForDimension1=[0 TV.LV.AMK.ID114 1000]  Table=[TV.LV.AMK.ID82*TV.LV.AMK.ID32771/100 TV.LV.AMK.ID82*TV.LV.AMK.ID32771/100 0]  InternalRulePriority=Speed  RndMeth=Simplest
  Max_Torque_Temperature_External_LUT : Lookup_n-D  NumberOfTableDimensions=1  BreakpointsForDimension1=[0 TV.LV.AMK.ID32798_11 TV.LV.AMK.ID32798_12]  Table=[TV.LV.AMK.ID82*TV.LV.AMK.ID32771/100 TV.LV.AMK.ID82*TV.LV.AMK.ID32771/100 0]  InternalRulePriority=Speed  RndMeth=Simplest
  Max_Torque_Temperature_IGBT_LUT : Lookup_n-D  NumberOfTableDimensions=1  BreakpointsForDimension1=[0 TV.LV.AMK.ID32798_8 TV.LV.AMK.ID32798_9]  Table=[TV.LV.AMK.ID82*TV.LV.AMK.ID32771/100 TV.LV.AMK.ID82*TV.LV.AMK.ID32771/100 0]  InternalRulePriority=Speed  RndMeth=Simplest
  Max_Torque_Temperature_Internal_LUT : Lookup_n-D  NumberOfTableDimensions=1  BreakpointsForDimension1=[0 TV.LV.AMK.ID32798_5 TV.LV.AMK.ID32798_6]  Table=[TV.LV.AMK.ID82*TV.LV.AMK.ID32771/100 TV.LV.AMK.ID82*TV.LV.AMK.ID32771/100 0]  InternalRulePriority=Speed  RndMeth=Simplest
  Min : MinMax  Inputs=7
  Mux : Mux
  Saturation_Positive : Saturate  UpperLimit=+inf  LowerLimit=0
  Torque_Curve : Subsystem
      mask Display: image('$imagefile'); % Use "Edit Image" on toolstrip to change.
  t_limit_positive : Outport
  wires:
  In Bus Element1/1 -> Cast_1/1  "display_overload_inverter"
  In Bus Element/1 -> Cast_0/1  "display_overload_motor"
  In Bus Element2/1 -> Cast_2/1  "temperature_internal"
  In Bus Element5/1 -> Torque_Curve/2(voltage [ID380])  "voltage"
  In Bus Element6/1 -> Torque_Curve/1(omega_wheels)  "omega_wheels"
  Max_Torque_Overload_Motor_LUT/1 -> Min/1  "max_torque_overload_motor"
  Max_Torque_Overload_Inverter_LUT/1 -> Min/2  "max_torque_overload_inverter_LUT"
  Max_Torque_Temperature_Internal_LUT/1 -> Min/3  "max_torque_temperature_internal"
  Max_Torque_Temperature_IGBT_LUT/1 -> Min/4  "max_torque_temperature_IGBT_LUT"
  In Bus torque_map1/1 -> Torque_Curve/3(torque_map)  "torque_map"
  Cast_0/1 -> Max_Torque_Overload_Motor_LUT/1
  Cast_1/1 -> Max_Torque_Overload_Inverter_LUT/1
  Cast_2/1 -> Max_Torque_Temperature_Internal_LUT/1
  Cast_3/1 -> Max_Torque_Temperature_IGBT_LUT/1
  Cast_4/1 -> Max_Torque_Temperature_External_LUT/1
  Min/1 -> Saturation_Positive/1  "t_limit"
  Max_Torque_Temperature_External_LUT/1 -> Min/5  "max_torque_temperature_external_LUT"
  Saturation_Positive/1 -> t_limit_positive/1  "t_limit_positive"
  Torque_Curve/1(max_torque_available) -> Min/6  "max_torque_available"
  Mux/1 -> Min/7
  Constant/1 -> Mux/1
  Constant1/1 -> Mux/2
  Constant2/1 -> Mux/3
  Constant3/1 -> Mux/4
  Constant4/1 -> Cast_3/1
  Constant5/1 -> Cast_4/1
